simulink model "Cascaded_FIR_filter"  (R2020b)
settings: Solver=VariableStepAuto  StartTime=0.0  StopTime=10.0  RelTol=1e-3
settings Model: Creator=hp  LastModifiedBy=hp
settings DataIOCC: SaveOutput=off  SaveTime=off

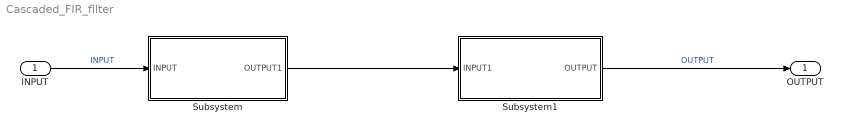
== system Cascaded_FIR_filter ==
  INPUT : Inport  OutDataTypeStr=double  PortDimensions=1  SampleTime=0
  Subsystem : Subsystem  TreatAsAtomicUnit=on
  Subsystem1 : Subsystem  TreatAsAtomicUnit=on
  OUTPUT : Outport  OutDataTypeStr=double  PortDimensions=1  SampleTime=0
  wires:
  INPUT/1 -> Subsystem/1(INPUT)  "INPUT"
  Subsystem/1(OUTPUT1) -> Subsystem1/1(INPUT1)
  Subsystem1/1(OUTPUT) -> OUTPUT/1  "OUTPUT"

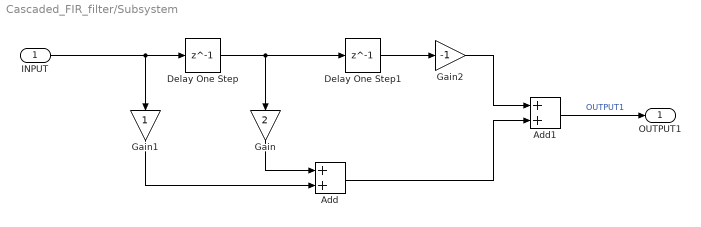
== system Cascaded_FIR_filter/Subsystem ==
  INPUT : Inport
  Add : Sum
  Add1 : Sum
  Delay One Step : Delay  DelayLength=1
  Delay One Step1 : Delay  DelayLength=1
  Gain : Gain  Gain=2
  Gain1 : Gain
  Gain2 : Gain  Gain=-1
  OUTPUT1 : Outport
  wires:
  Add1/1 -> OUTPUT1/1  "OUTPUT1"
  Gain1/1 -> Add/2
  Delay One Step/1 -> Gain/1, Delay One Step1/1
  INPUT/1 -> Gain1/1, Delay One Step/1
  Add/1 -> Add1/2
  Gain2/1 -> Add1/1
  Gain/1 -> Add/1
  Delay One Step1/1 -> Gain2/1

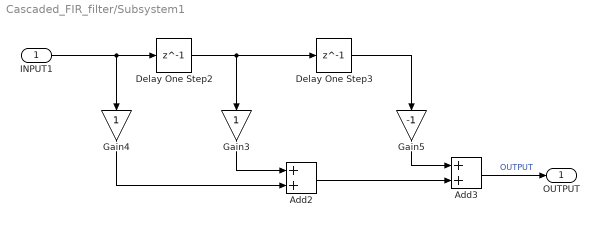
== system Cascaded_FIR_filter/Subsystem1 ==
  INPUT1 : Inport
  Add2 : Sum
  Add3 : Sum
  Delay One Step2 : Delay  DelayLength=1
  Delay One Step3 : Delay  DelayLength=1
  Gain3 : Gain
  Gain4 : Gain
  Gain5 : Gain  Gain=-1
  OUTPUT : Outport
  wires:
  Delay One Step3/1 -> Gain5/1
  Gain3/1 -> Add2/1
  Add3/1 -> OUTPUT/1  "OUTPUT"
  Add2/1 -> Add3/2
  Delay One Step2/1 -> Gain3/1, Delay One Step3/1
  Gain4/1 -> Add2/2
  INPUT1/1 -> Delay One Step2/1, Gain4/1
  Gain5/1 -> Add3/1
